simulink model "Mathmatical_Equation_S_Domain"  (R2023a)
settings: Solver=VariableStepAuto  StartTime=0.0  StopTime=50  MaxStep=0.01  RelTol=1e-3
values from neighbouring files (symbols this model uses):
  b = 0.5    [Mathmatical_Equation_S_Domain_script.m]
  k = 10    [Mathmatical_Equation_S_Domain_script.m]
  M = 1    [Mathmatical_Equation_S_Domain_script.m]
libraries: dspsrcs4 x1
settings Model: Creator=ass1728  LastModifiedBy=ass1728

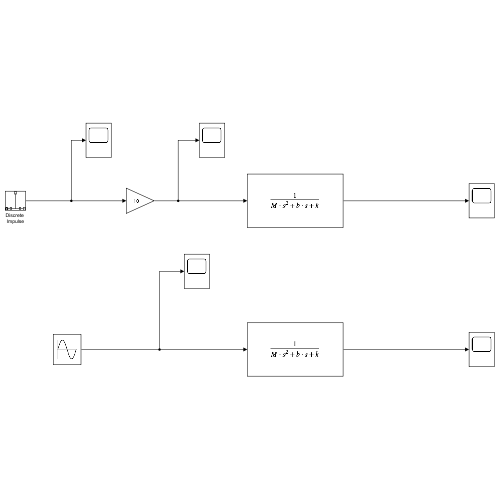
[thumbnail: Simulink's stored preview of the top-level diagram]
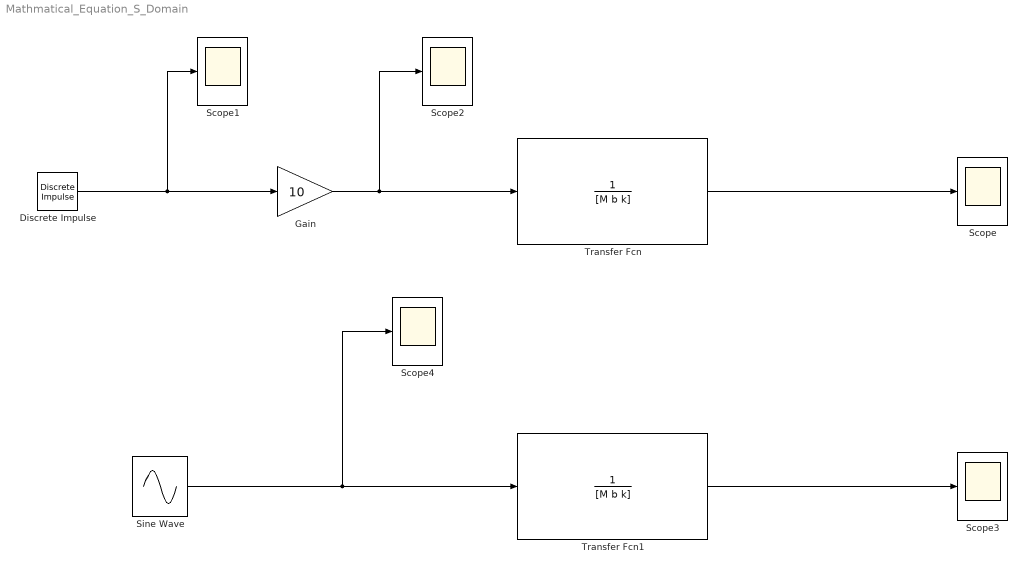
== system Mathmatical_Equation_S_Domain ==
  Discrete Impulse : dspsrcs4/Discrete  Impulse  Delay=0  SampleTime=1  FrameSample=1  OutputFrames=off  dataType=double  isSigned=on  wordLen=16  udDataType=sfix(16)  fracBitsMode=Best precision  numFracBits=15  OutDataTypeStr=double  LastOutDataTypeStr=double
  Gain : Gain  Gain=10
  Scope{,1..4} (5 alike) : Scope
  Sine Wave : Sin  SampleTime=0
  Transfer Fcn : TransferFcn  Denominator=[M b k]
  Transfer Fcn1 : TransferFcn  Denominator=[M b k]
  wires:
  Transfer Fcn/1 -> Scope/1
  Discrete Impulse/1 -> Scope1/1, Gain/1
  Gain/1 -> Scope2/1, Transfer Fcn/1
  Transfer Fcn1/1 -> Scope3/1
  Sine Wave/1 -> Scope4/1, Transfer Fcn1/1
